simulink model "tf_est"  (R2014a)
settings: Solver=ode45  StartTime=0.0  StopTime=10.0  FixedStep=0.01  RelTol=1e-3
libraries: cstblocks x1
settings Model: Creator=Gracex  LastModifiedBy=Gracex
settings DebuggingCC: SolverPrmCheckMsg=none

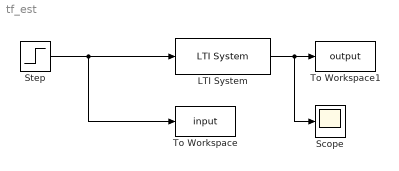
== system tf_est ==
  LTI System : cstblocks/LTI System  sys=G_s  IC=[]
  Scope : Scope
  Step : Step  SampleTime=0
  To Workspace : ToWorkspace  VariableName=input  SampleTime=-1
      settings: Save2DSignal=2-D array (concatenate along first dimension)
  To Workspace1 : ToWorkspace  VariableName=output  SampleTime=-1
      settings: Save2DSignal=2-D array (concatenate along first dimension)
  wires:
  LTI System/1 -> Scope/1, To Workspace1/1
  Step/1 -> LTI System/1, To Workspace/1
